simulink model "LMS_cs"  (R2023a)
settings: Solver=ode5  StartTime=0.0  StopTime=inf  FixedStep=1/200  RelTol=1e-3
PreLoadFcn:
  | mbxruntime.callbacks.PreLoadFcn(bdroot);
PostLoadFcn:
  | mbxruntime.callbacks.PostLoadFcn(bdroot);
InitFcn:
  | mbxruntime.callbacks.InitFcn(bdroot);
StartFcn:
  | mbxruntime.callbacks.StartFcn(bdroot);
StopFcn:
  | mbxruntime.callbacks.StopFcn(bdroot);
model workspace (MAT data in the model file):
  mbox_table : object (value not decoded)
  model_closed = 0
  sim_status = 0
undefined symbols (not defined in the file or in its folder): DiscIntNeverNeededParam, WheelL0, WheelL1, WheelR0, WheelR1
libraries: simulink x462, simulink_extras x117, PreScanSimulinkLibrary x33, PreScanUsefulBlocks x6, instrumentseriallib x5, simulink_need_slupdate x1
(part 66 of 68)

== system LMS_cs/BMW_X5_SUV_3/Dynamics_Simple_3D/Chassis/Bicycle_model_[XYZ]/RoadContact/RoadGeometry/zRR_lowerpenetrationdetph ==
  penetrationdepth : Inport
  position_z : Inport  Port=2
  normal_z : Inport  Port=3
  Add : Sum  Inputs=-+
  Configurable Subsystem : Subsystem  BlockChoice=Transfer Fcn  mask{ComputationMode=ComputationMode}
      mask prompts: ComputationMode "Compuation mode:"
      mask init:
      | SetComputationMode(gcb,ComputationMode);
      settings: AttributesFormatString=%<BlockChoice>  OpenFcn=BringToFront(gcb);  MemberBlocks=Discrete Transfer Fcn,Transfer Fcn
      settings: TemplateBlock=|
      | PreScanSimulinkLibrary/Configurable Subsystems/TransferFunction
      | lowerpenetrationdetph/Configurable
      | Subsystem
  Constant : Constant  Value=Inf
  Constant1 : Constant  Value=-6
  Constant2 : Constant  Value=-Inf
  Data Type Conversion : DataTypeConversion  OutDataTypeStr=double  SaturateOnIntegerOverflow=off  RndMeth=Floor
  MinMax : MinMax
  Product : Product  RndMeth=Zero
  Product1 : Product  Inputs=/*  RndMeth=Zero
  Product2 : Product  RndMeth=Zero
  Rate Limiter Dynamic : simulink/Discontinuities/Rate Limiter Dynamic
  Relational Operator : RelationalOperator  Operator===  OutDataTypeStr=boolean  InputSameDT=off
  Sum of Elements : Sum  Inputs=+
  Sum of Elements1 : Sum  Inputs=+
  Sum of Elements2 : Sum  Inputs=+
  Switch : Switch  SaturateOnIntegerOverflow=off  InputSameDT=off
  z : Outport
  wires:
  Configurable Subsystem/1(Out1) -> z/1
  Rate Limiter Dynamic/1 -> Configurable Subsystem/1(In1)
  Switch/1 -> Rate Limiter Dynamic/3
  Constant2/1 -> Switch/3
  Constant1/1 -> Switch/1
  Sum of Elements2/1 -> Switch/2
  Constant/1 -> Rate Limiter Dynamic/1
  Product1/1 -> Rate Limiter Dynamic/2
  position_z/1 -> Add/2
  Product2/1 -> Add/1
  Sum of Elements/1 -> Product1/2
  Sum of Elements1/1 -> Product1/1
  Relational Operator/1 -> Data Type Conversion/1
  Product/1 -> Sum of Elements/1
  MinMax/1 -> Relational Operator/2
  penetrationdepth/1 -> Sum of Elements2/1, Relational Operator/1, MinMax/1, Product2/1
  Add/1 -> Product/2
  normal_z/1 -> Product2/2
  Data Type Conversion/1 -> Sum of Elements1/1, Product/1

== system LMS_cs/BMW_X5_SUV_3/Dynamics_Simple_3D/Chassis/Bicycle_model_[XYZ]/RoadContact/RoadGeometry/zRR_tyreinfo ==
  In1 : Inport
  Bus Selector2 : BusSelector  OutputSignals=TireRR.cp0.penetrationdepth,TireRR.cp1.penetrationdepth,TireRR.cp2.penetrationdepth,TireRR.cp3.penetrationdepth,TireRR.cp0.position.z,TireRR.cp1.position.z,TireRR.cp2.position.z,TireRR.cp3.position.z,TireRR.cp0.normal.z,TireRR.cp1.normal.z,TireRR.cp2.normal.z,TireRR.cp3.normal.z
  Mux11 : Mux
  Mux12 : Mux
  Mux13 : Mux
  penetrationdepth : Outport
  position_z : Outport  Port=2
  normal_z : Outport  Port=3
  wires:
  Mux13/1 -> normal_z/1
  Mux12/1 -> position_z/1
  Mux11/1 -> penetrationdepth/1
  In1/1 -> Bus Selector2/1
  Bus Selector2/12 -> Mux13/4  "<z>"
  Bus Selector2/11 -> Mux13/3  "<z>"
  Bus Selector2/10 -> Mux13/2  "<z>"
  Bus Selector2/9 -> Mux13/1  "<z>"
  Bus Selector2/8 -> Mux12/4  "<z>"
  Bus Selector2/7 -> Mux12/3  "<z>"
  Bus Selector2/6 -> Mux12/2  "<z>"
  Bus Selector2/5 -> Mux12/1  "<z>"
  Bus Selector2/4 -> Mux11/4  "<penetrationdepth>"
  Bus Selector2/3 -> Mux11/3  "<penetrationdepth>"
  Bus Selector2/2 -> Mux11/2  "<penetrationdepth>"
  Bus Selector2/1 -> Mux11/1  "<penetrationdepth>"

== system LMS_cs/BMW_X5_SUV_3/Dynamics_Simple_3D/Chassis/Bicycle_model_[XYZ]/X_Motion/Max RPM and zero- velocity detection/Configurable Subsystem ==
  Step : Step  Time=0.0001  Before=1  After=0  SampleTime=0
  Out1 : Outport
  wires:
  Step/1 -> Out1/1

== system LMS_cs/BMW_X5_SUV_3/Dynamics_Simple_3D/Chassis/Bicycle_model_[XYZ]/X_Motion/Max RPM and zero- velocity detection/SR-Memory ==
  Signal : Inport
  Set : Inport  Port=2
  Reset : Inport  Port=3
  Constant : Constant  Value=0
  Detect Rise Positive : simulink/Logic and Bit Operations/Detect Rise Positive  vinit=0  OutDataTypeStr=uint8
  Detect Rise Positive1 : simulink/Logic and Bit Operations/Detect Rise Positive  vinit=0  OutDataTypeStr=uint8
  Manual Switch : ManualSwitch
  Manual Switch1 : ManualSwitch
  Switch : Switch  Criteria=u2 ~= 0  SaturateOnIntegerOverflow=off  InputSameDT=off
  Switch1 : Switch  Criteria=u2 ~= 0  SaturateOnIntegerOverflow=off  InputSameDT=off
  Unit Delay : UnitDelay  SampleTime=-1  HasFrameUpgradeWarning=on
  Out : Outport
  wires:
  Manual Switch/1 -> Switch/2
  Detect Rise Positive/1 -> Manual Switch/1
  Set/1 -> Manual Switch/2, Detect Rise Positive/1
  Unit Delay/1 -> Switch/3
  Signal/1 -> Switch/1
  Detect Rise Positive1/1 -> Manual Switch1/1
  Reset/1 -> Detect Rise Positive1/1, Manual Switch1/2
  Manual Switch1/1 -> Switch1/2
  Switch1/1 -> Out/1, Unit Delay/1
  Switch/1 -> Switch1/3
  Constant/1 -> Switch1/1

== system LMS_cs/BMW_X5_SUV_3/PreScan_Contact_Sensor/Vehicle Local to World/state2FullState/limit roll/Substitute 90 & 270 deg (and its plurals)/Angle 0-360 deg limiter ==
  Angle [deg] : Inport
  Gain : Gain  Gain=1/360
  Gain1 : Gain  Gain=360
  Rounding Function : Rounding
  Sum : Sum  Inputs=|-+
  LimAngle [deg] : Outport
  wires:
  Gain/1 -> Rounding Function/1
  Rounding Function/1 -> Gain1/1
  Gain1/1 -> Sum/1
  Angle [deg]/1 -> Gain/1, Sum/2
  Sum/1 -> LimAngle [deg]/1

== system LMS_cs/BMW_X5_SUV_4/Dynamics_Simple_3D/Chassis/Bicycle_model_[XYZ]/RoadContact/RoadGeometry/Calc_banking ==
  zi : Inport
  Constant : Constant  Value=[1, -1, 1, -1]
  Gain : Gain  Gain=1/(p.width*2)
  Product : Product  RndMeth=Zero
  Saturation : Saturate  UpperLimit=1  LowerLimit=-1
  Sum of Elements : Sum  Inputs=+
  Trigonometric Function : Trigonometry  Operator=asin
  banking : Outport
  wires:
  Saturation/1 -> Trigonometric Function/1
  zi/1 -> Product/1
  Constant/1 -> Product/2
  Product/1 -> Sum of Elements/1
  Gain/1 -> Saturation/1
  Sum of Elements/1 -> Gain/1
  Trigonometric Function/1 -> banking/1

== system LMS_cs/BMW_X5_SUV_4/Dynamics_Simple_3D/Chassis/Bicycle_model_[XYZ]/RoadContact/RoadGeometry/Calc_slope ==
  zi : Inport
  Constant : Constant  Value=[-1, -1, 1, 1]
  Gain : Gain  Gain=1/(p.l*2)
  Product : Product  RndMeth=Zero
  Saturation : Saturate  UpperLimit=1  LowerLimit=-1
  Sum of Elements : Sum  Inputs=+
  Trigonometric Function : Trigonometry  Operator=asin
  slope : Outport
  wires:
  Saturation/1 -> Trigonometric Function/1
  zi/1 -> Product/1
  Constant/1 -> Product/2
  Product/1 -> Sum of Elements/1
  Gain/1 -> Saturation/1
  Sum of Elements/1 -> Gain/1
  Trigonometric Function/1 -> slope/1

== system LMS_cs/BMW_X5_SUV_4/Dynamics_Simple_3D/Chassis/Bicycle_model_[XYZ]/RoadContact/RoadGeometry/Calc_z ==
  zi : Inport
  zC : Subsystem
  z : Outport
  wires:
  zC/1(Mean) -> z/1
  zi/1 -> zC/1(Array)

== system LMS_cs/BMW_X5_SUV_4/Dynamics_Simple_3D/Chassis/Bicycle_model_[XYZ]/RoadContact/RoadGeometry/zFL_lowerpenetrationdetph ==
  penetrationdepth : Inport
  position_z : Inport  Port=2
  normal_z : Inport  Port=3
  Add : Sum  Inputs=-+
  Configurable Subsystem : Subsystem  BlockChoice=Transfer Fcn  mask{ComputationMode=ComputationMode}
      mask prompts: ComputationMode "Compuation mode:"
      mask init:
      | SetComputationMode(gcb,ComputationMode);
      settings: AttributesFormatString=%<BlockChoice>  OpenFcn=BringToFront(gcb);  MemberBlocks=Discrete Transfer Fcn,Transfer Fcn
      settings: TemplateBlock=|
      | PreScanSimulinkLibrary/Configurable Subsystems/TransferFunction
      | lowerpenetrationdetph/Configurable
      | Subsystem
  Constant : Constant  Value=Inf
  Constant1 : Constant  Value=-6
  Constant2 : Constant  Value=-Inf
  Data Type Conversion : DataTypeConversion  OutDataTypeStr=double  SaturateOnIntegerOverflow=off  RndMeth=Floor
  MinMax : MinMax
  Product : Product  RndMeth=Zero
  Product1 : Product  Inputs=/*  RndMeth=Zero
  Product2 : Product  RndMeth=Zero
  Rate Limiter Dynamic : simulink/Discontinuities/Rate Limiter Dynamic
  Relational Operator : RelationalOperator  Operator===  OutDataTypeStr=boolean  InputSameDT=off
  Sum of Elements : Sum  Inputs=+
  Sum of Elements1 : Sum  Inputs=+
  Sum of Elements2 : Sum  Inputs=+
  Switch : Switch  SaturateOnIntegerOverflow=off  InputSameDT=off
  z : Outport
  wires:
  normal_z/1 -> Product2/2
  Add/1 -> Product/2
  penetrationdepth/1 -> Product2/1, MinMax/1, Relational Operator/1, Sum of Elements2/1
  MinMax/1 -> Relational Operator/2
  Product/1 -> Sum of Elements/1
  Relational Operator/1 -> Data Type Conversion/1
  Sum of Elements1/1 -> Product1/1
  Sum of Elements/1 -> Product1/2
  Product2/1 -> Add/1
  position_z/1 -> Add/2
  Product1/1 -> Rate Limiter Dynamic/2
  Constant/1 -> Rate Limiter Dynamic/1
  Sum of Elements2/1 -> Switch/2
  Constant1/1 -> Switch/1
  Constant2/1 -> Switch/3
  Switch/1 -> Rate Limiter Dynamic/3
  Rate Limiter Dynamic/1 -> Configurable Subsystem/1(In1)
  Configurable Subsystem/1(Out1) -> z/1
  Data Type Conversion/1 -> Product/1, Sum of Elements1/1

== system LMS_cs/BMW_X5_SUV_4/Dynamics_Simple_3D/Chassis/Bicycle_model_[XYZ]/RoadContact/RoadGeometry/zFL_tyreinfo ==
  In1 : Inport
  Bus Selector2 : BusSelector  OutputSignals=TireFL.cp0.penetrationdepth,TireFL.cp1.penetrationdepth,TireFL.cp2.penetrationdepth,TireFL.cp3.penetrationdepth,TireFL.cp0.position.z,TireFL.cp1.position.z,TireFL.cp2.position.z,TireFL.cp3.position.z,TireFL.cp0.normal.z,TireFL.cp1.normal.z,TireFL.cp2.normal.z,TireFL.cp3.normal.z
  Mux11 : Mux
  Mux12 : Mux
  Mux13 : Mux
  penetrationdepth : Outport
  position_z : Outport  Port=2
  normal_z : Outport  Port=3
  wires:
  Bus Selector2/1 -> Mux11/1  "<penetrationdepth>"
  Bus Selector2/2 -> Mux11/2  "<penetrationdepth>"
  Bus Selector2/3 -> Mux11/3  "<penetrationdepth>"
  Bus Selector2/4 -> Mux11/4  "<penetrationdepth>"
  Bus Selector2/5 -> Mux12/1  "<z>"
  Bus Selector2/6 -> Mux12/2  "<z>"
  Bus Selector2/7 -> Mux12/3  "<z>"
  Bus Selector2/8 -> Mux12/4  "<z>"
  Bus Selector2/9 -> Mux13/1  "<z>"
  Bus Selector2/10 -> Mux13/2  "<z>"
  Bus Selector2/11 -> Mux13/3  "<z>"
  Bus Selector2/12 -> Mux13/4  "<z>"
  In1/1 -> Bus Selector2/1
  Mux11/1 -> penetrationdepth/1
  Mux12/1 -> position_z/1
  Mux13/1 -> normal_z/1

== system LMS_cs/BMW_X5_SUV_4/Dynamics_Simple_3D/Chassis/Bicycle_model_[XYZ]/RoadContact/RoadGeometry/zFR_lowerpenetrationdetph ==
  penetrationdepth : Inport
  position_z : Inport  Port=2
  normal_z : Inport  Port=3
  Add : Sum  Inputs=-+
  Configurable Subsystem : Subsystem  BlockChoice=Transfer Fcn  mask{ComputationMode=ComputationMode}
      mask prompts: ComputationMode "Compuation mode:"
      mask init:
      | SetComputationMode(gcb,ComputationMode);
      settings: AttributesFormatString=%<BlockChoice>  OpenFcn=BringToFront(gcb);  MemberBlocks=Discrete Transfer Fcn,Transfer Fcn
      settings: TemplateBlock=|
      | PreScanSimulinkLibrary/Configurable Subsystems/TransferFunction
      | lowerpenetrationdetph/Configurable
      | Subsystem
  Constant : Constant  Value=Inf
  Constant1 : Constant  Value=-6
  Constant2 : Constant  Value=-Inf
  Data Type Conversion : DataTypeConversion  OutDataTypeStr=double  SaturateOnIntegerOverflow=off  RndMeth=Floor
  MinMax : MinMax
  Product : Product  RndMeth=Zero
  Product1 : Product  Inputs=/*  RndMeth=Zero
  Product2 : Product  RndMeth=Zero
  Rate Limiter Dynamic : simulink/Discontinuities/Rate Limiter Dynamic
  Relational Operator : RelationalOperator  Operator===  OutDataTypeStr=boolean  InputSameDT=off
  Sum of Elements : Sum  Inputs=+
  Sum of Elements1 : Sum  Inputs=+
  Sum of Elements2 : Sum  Inputs=+
  Switch : Switch  SaturateOnIntegerOverflow=off  InputSameDT=off
  z : Outport
  wires:
  Configurable Subsystem/1(Out1) -> z/1
  Rate Limiter Dynamic/1 -> Configurable Subsystem/1(In1)
  Switch/1 -> Rate Limiter Dynamic/3
  Constant2/1 -> Switch/3
  Constant1/1 -> Switch/1
  Sum of Elements2/1 -> Switch/2
  Constant/1 -> Rate Limiter Dynamic/1
  Product1/1 -> Rate Limiter Dynamic/2
  position_z/1 -> Add/2
  Product2/1 -> Add/1
  Sum of Elements/1 -> Product1/2
  Sum of Elements1/1 -> Product1/1
  Relational Operator/1 -> Data Type Conversion/1
  Product/1 -> Sum of Elements/1
  MinMax/1 -> Relational Operator/2
  penetrationdepth/1 -> Sum of Elements2/1, Relational Operator/1, MinMax/1, Product2/1
  Add/1 -> Product/2
  normal_z/1 -> Product2/2
  Data Type Conversion/1 -> Sum of Elements1/1, Product/1

== system LMS_cs/BMW_X5_SUV_4/Dynamics_Simple_3D/Chassis/Bicycle_model_[XYZ]/RoadContact/RoadGeometry/zFR_tyreinfo ==
  In1 : Inport
  Bus Selector2 : BusSelector  OutputSignals=TireFR.cp0.penetrationdepth,TireFR.cp1.penetrationdepth,TireFR.cp2.penetrationdepth,TireFR.cp3.penetrationdepth,TireFR.cp0.position.z,TireFR.cp1.position.z,TireFR.cp2.position.z,TireFR.cp3.position.z,TireFR.cp0.normal.z,TireFR.cp1.normal.z,TireFR.cp2.normal.z,TireFR.cp3.normal.z
  Mux11 : Mux
  Mux12 : Mux
  Mux13 : Mux
  penetrationdepth : Outport
  position_z : Outport  Port=2
  normal_z : Outport  Port=3
  wires:
  Mux13/1 -> normal_z/1
  Mux12/1 -> position_z/1
  Mux11/1 -> penetrationdepth/1
  In1/1 -> Bus Selector2/1
  Bus Selector2/12 -> Mux13/4  "<z>"
  Bus Selector2/11 -> Mux13/3  "<z>"
  Bus Selector2/10 -> Mux13/2  "<z>"
  Bus Selector2/9 -> Mux13/1  "<z>"
  Bus Selector2/8 -> Mux12/4  "<z>"
  Bus Selector2/7 -> Mux12/3  "<z>"
  Bus Selector2/6 -> Mux12/2  "<z>"
  Bus Selector2/5 -> Mux12/1  "<z>"
  Bus Selector2/4 -> Mux11/4  "<penetrationdepth>"
  Bus Selector2/3 -> Mux11/3  "<penetrationdepth>"
  Bus Selector2/2 -> Mux11/2  "<penetrationdepth>"
  Bus Selector2/1 -> Mux11/1  "<penetrationdepth>"

== system LMS_cs/BMW_X5_SUV_4/Dynamics_Simple_3D/Chassis/Bicycle_model_[XYZ]/RoadContact/RoadGeometry/zRL_lowerpenetrationdetph ==
  penetrationdepth : Inport
  position_z : Inport  Port=2
  normal_z : Inport  Port=3
  Add : Sum  Inputs=-+
  Configurable Subsystem : Subsystem  BlockChoice=Transfer Fcn  mask{ComputationMode=ComputationMode}
      mask prompts: ComputationMode "Compuation mode:"
      mask init:
      | SetComputationMode(gcb,ComputationMode);
      settings: AttributesFormatString=%<BlockChoice>  OpenFcn=BringToFront(gcb);  MemberBlocks=Discrete Transfer Fcn,Transfer Fcn
      settings: TemplateBlock=|
      | PreScanSimulinkLibrary/Configurable Subsystems/TransferFunction
      | lowerpenetrationdetph/Configurable
      | Subsystem
  Constant : Constant  Value=Inf
  Constant1 : Constant  Value=-6
  Constant2 : Constant  Value=-Inf
  Data Type Conversion : DataTypeConversion  OutDataTypeStr=double  SaturateOnIntegerOverflow=off  RndMeth=Floor
  MinMax : MinMax
  Product : Product  RndMeth=Zero
  Product1 : Product  Inputs=/*  RndMeth=Zero
  Product2 : Product  RndMeth=Zero
  Rate Limiter Dynamic : simulink/Discontinuities/Rate Limiter Dynamic
  Relational Operator : RelationalOperator  Operator===  OutDataTypeStr=boolean  InputSameDT=off
  Sum of Elements : Sum  Inputs=+
  Sum of Elements1 : Sum  Inputs=+
  Sum of Elements2 : Sum  Inputs=+
  Switch : Switch  SaturateOnIntegerOverflow=off  InputSameDT=off
  z : Outport
  wires:
  normal_z/1 -> Product2/2
  Add/1 -> Product/2
  penetrationdepth/1 -> Product2/1, MinMax/1, Relational Operator/1, Sum of Elements2/1
  MinMax/1 -> Relational Operator/2
  Product/1 -> Sum of Elements/1
  Relational Operator/1 -> Data Type Conversion/1
  Sum of Elements1/1 -> Product1/1
  Sum of Elements/1 -> Product1/2
  Product2/1 -> Add/1
  position_z/1 -> Add/2
  Product1/1 -> Rate Limiter Dynamic/2
  Constant/1 -> Rate Limiter Dynamic/1
  Sum of Elements2/1 -> Switch/2
  Constant1/1 -> Switch/1
  Constant2/1 -> Switch/3
  Switch/1 -> Rate Limiter Dynamic/3
  Rate Limiter Dynamic/1 -> Configurable Subsystem/1(In1)
  Configurable Subsystem/1(Out1) -> z/1
  Data Type Conversion/1 -> Product/1, Sum of Elements1/1

== system LMS_cs/BMW_X5_SUV_4/Dynamics_Simple_3D/Chassis/Bicycle_model_[XYZ]/RoadContact/RoadGeometry/zRL_tyreinfo ==
  In1 : Inport
  Bus Selector2 : BusSelector  OutputSignals=TireRL.cp0.penetrationdepth,TireRL.cp1.penetrationdepth,TireRL.cp2.penetrationdepth,TireRL.cp3.penetrationdepth,TireRL.cp0.position.z,TireRL.cp1.position.z,TireRL.cp2.position.z,TireRL.cp3.position.z,TireRL.cp0.normal.z,TireRL.cp1.normal.z,TireRL.cp2.normal.z,TireRL.cp3.normal.z
  Mux11 : Mux
  Mux12 : Mux
  Mux13 : Mux
  penetrationdepth : Outport
  position_z : Outport  Port=2
  normal_z : Outport  Port=3
  wires:
  Bus Selector2/1 -> Mux11/1  "<penetrationdepth>"
  Bus Selector2/2 -> Mux11/2  "<penetrationdepth>"
  Bus Selector2/3 -> Mux11/3  "<penetrationdepth>"
  Bus Selector2/4 -> Mux11/4  "<penetrationdepth>"
  Bus Selector2/5 -> Mux12/1  "<z>"
  Bus Selector2/6 -> Mux12/2  "<z>"
  Bus Selector2/7 -> Mux12/3  "<z>"
  Bus Selector2/8 -> Mux12/4  "<z>"
  Bus Selector2/9 -> Mux13/1  "<z>"
  Bus Selector2/10 -> Mux13/2  "<z>"
  Bus Selector2/11 -> Mux13/3  "<z>"
  Bus Selector2/12 -> Mux13/4  "<z>"
  In1/1 -> Bus Selector2/1
  Mux11/1 -> penetrationdepth/1
  Mux12/1 -> position_z/1
  Mux13/1 -> normal_z/1

== system LMS_cs/BMW_X5_SUV_4/Dynamics_Simple_3D/Chassis/Bicycle_model_[XYZ]/RoadContact/RoadGeometry/zRR_lowerpenetrationdetph ==
  penetrationdepth : Inport
  position_z : Inport  Port=2
  normal_z : Inport  Port=3
  Add : Sum  Inputs=-+
  Configurable Subsystem : Subsystem  BlockChoice=Transfer Fcn  mask{ComputationMode=ComputationMode}
      mask prompts: ComputationMode "Compuation mode:"
      mask init:
      | SetComputationMode(gcb,ComputationMode);
      settings: AttributesFormatString=%<BlockChoice>  OpenFcn=BringToFront(gcb);  MemberBlocks=Discrete Transfer Fcn,Transfer Fcn
      settings: TemplateBlock=|
      | PreScanSimulinkLibrary/Configurable Subsystems/TransferFunction
      | lowerpenetrationdetph/Configurable
      | Subsystem
  Constant : Constant  Value=Inf
  Constant1 : Constant  Value=-6
  Constant2 : Constant  Value=-Inf
  Data Type Conversion : DataTypeConversion  OutDataTypeStr=double  SaturateOnIntegerOverflow=off  RndMeth=Floor
  MinMax : MinMax
  Product : Product  RndMeth=Zero
  Product1 : Product  Inputs=/*  RndMeth=Zero
  Product2 : Product  RndMeth=Zero
  Rate Limiter Dynamic : simulink/Discontinuities/Rate Limiter Dynamic
  Relational Operator : RelationalOperator  Operator===  OutDataTypeStr=boolean  InputSameDT=off
  Sum of Elements : Sum  Inputs=+
  Sum of Elements1 : Sum  Inputs=+
  Sum of Elements2 : Sum  Inputs=+
  Switch : Switch  SaturateOnIntegerOverflow=off  InputSameDT=off
  z : Outport
  wires:
  Configurable Subsystem/1(Out1) -> z/1
  Rate Limiter Dynamic/1 -> Configurable Subsystem/1(In1)
  Switch/1 -> Rate Limiter Dynamic/3
  Constant2/1 -> Switch/3
  Constant1/1 -> Switch/1
  Sum of Elements2/1 -> Switch/2
  Constant/1 -> Rate Limiter Dynamic/1
  Product1/1 -> Rate Limiter Dynamic/2
  position_z/1 -> Add/2
  Product2/1 -> Add/1
  Sum of Elements/1 -> Product1/2
  Sum of Elements1/1 -> Product1/1
  Relational Operator/1 -> Data Type Conversion/1
  Product/1 -> Sum of Elements/1
  MinMax/1 -> Relational Operator/2
  penetrationdepth/1 -> Sum of Elements2/1, Relational Operator/1, MinMax/1, Product2/1
  Add/1 -> Product/2
  normal_z/1 -> Product2/2
  Data Type Conversion/1 -> Sum of Elements1/1, Product/1

== system LMS_cs/BMW_X5_SUV_4/Dynamics_Simple_3D/Chassis/Bicycle_model_[XYZ]/RoadContact/RoadGeometry/zRR_tyreinfo ==
  In1 : Inport
  Bus Selector2 : BusSelector  OutputSignals=TireRR.cp0.penetrationdepth,TireRR.cp1.penetrationdepth,TireRR.cp2.penetrationdepth,TireRR.cp3.penetrationdepth,TireRR.cp0.position.z,TireRR.cp1.position.z,TireRR.cp2.position.z,TireRR.cp3.position.z,TireRR.cp0.normal.z,TireRR.cp1.normal.z,TireRR.cp2.normal.z,TireRR.cp3.normal.z
  Mux11 : Mux
  Mux12 : Mux
  Mux13 : Mux
  penetrationdepth : Outport
  position_z : Outport  Port=2
  normal_z : Outport  Port=3
  wires:
  Mux13/1 -> normal_z/1
  Mux12/1 -> position_z/1
  Mux11/1 -> penetrationdepth/1
  In1/1 -> Bus Selector2/1
  Bus Selector2/12 -> Mux13/4  "<z>"
  Bus Selector2/11 -> Mux13/3  "<z>"
  Bus Selector2/10 -> Mux13/2  "<z>"
  Bus Selector2/9 -> Mux13/1  "<z>"
  Bus Selector2/8 -> Mux12/4  "<z>"
  Bus Selector2/7 -> Mux12/3  "<z>"
  Bus Selector2/6 -> Mux12/2  "<z>"
  Bus Selector2/5 -> Mux12/1  "<z>"
  Bus Selector2/4 -> Mux11/4  "<penetrationdepth>"
  Bus Selector2/3 -> Mux11/3  "<penetrationdepth>"
  Bus Selector2/2 -> Mux11/2  "<penetrationdepth>"
  Bus Selector2/1 -> Mux11/1  "<penetrationdepth>"

== system LMS_cs/BMW_X5_SUV_4/Dynamics_Simple_3D/Chassis/Bicycle_model_[XYZ]/X_Motion/Max RPM and zero- velocity detection/Configurable Subsystem ==
  Step : Step  Time=0.0001  Before=1  After=0  SampleTime=0
  Out1 : Outport
  wires:
  Step/1 -> Out1/1

== system LMS_cs/BMW_X5_SUV_4/Dynamics_Simple_3D/Chassis/Bicycle_model_[XYZ]/X_Motion/Max RPM and zero- velocity detection/SR-Memory ==
  Signal : Inport
  Set : Inport  Port=2
  Reset : Inport  Port=3
  Constant : Constant  Value=0
  Detect Rise Positive : simulink/Logic and Bit Operations/Detect Rise Positive  vinit=0  OutDataTypeStr=uint8
  Detect Rise Positive1 : simulink/Logic and Bit Operations/Detect Rise Positive  vinit=0  OutDataTypeStr=uint8
  Manual Switch : ManualSwitch
  Manual Switch1 : ManualSwitch
  Switch : Switch  Criteria=u2 ~= 0  SaturateOnIntegerOverflow=off  InputSameDT=off
  Switch1 : Switch  Criteria=u2 ~= 0  SaturateOnIntegerOverflow=off  InputSameDT=off
  Unit Delay : UnitDelay  SampleTime=-1  HasFrameUpgradeWarning=on
  Out : Outport
  wires:
  Manual Switch/1 -> Switch/2
  Detect Rise Positive/1 -> Manual Switch/1
  Set/1 -> Manual Switch/2, Detect Rise Positive/1
  Unit Delay/1 -> Switch/3
  Signal/1 -> Switch/1
  Detect Rise Positive1/1 -> Manual Switch1/1
  Reset/1 -> Detect Rise Positive1/1, Manual Switch1/2
  Manual Switch1/1 -> Switch1/2
  Switch1/1 -> Out/1, Unit Delay/1
  Switch/1 -> Switch1/3
  Constant/1 -> Switch1/1

== system LMS_cs/BMW_X5_SUV_4/PreScan_Contact_Sensor/Vehicle Local to World/state2FullState/limit roll/Substitute 90 & 270 deg (and its plurals)/Angle 0-360 deg limiter ==
  Angle [deg] : Inport
  Gain : Gain  Gain=1/360
  Gain1 : Gain  Gain=360
  Rounding Function : Rounding
  Sum : Sum  Inputs=|-+
  LimAngle [deg] : Outport
  wires:
  Gain/1 -> Rounding Function/1
  Rounding Function/1 -> Gain1/1
  Gain1/1 -> Sum/1
  Angle [deg]/1 -> Gain/1, Sum/2
  Sum/1 -> LimAngle [deg]/1

== system LMS_cs/BMW_X5_SUV_5/Dynamics_Simple_3D/Chassis/Bicycle_model_[XYZ]/RoadContact/RoadGeometry/Calc_banking ==
  zi : Inport
  Constant : Constant  Value=[1, -1, 1, -1]
  Gain : Gain  Gain=1/(p.width*2)
  Product : Product  RndMeth=Zero
  Saturation : Saturate  UpperLimit=1  LowerLimit=-1
  Sum of Elements : Sum  Inputs=+
  Trigonometric Function : Trigonometry  Operator=asin
  banking : Outport
  wires:
  Saturation/1 -> Trigonometric Function/1
  zi/1 -> Product/1
  Constant/1 -> Product/2
  Product/1 -> Sum of Elements/1
  Gain/1 -> Saturation/1
  Sum of Elements/1 -> Gain/1
  Trigonometric Function/1 -> banking/1

== system LMS_cs/BMW_X5_SUV_5/Dynamics_Simple_3D/Chassis/Bicycle_model_[XYZ]/RoadContact/RoadGeometry/Calc_slope ==
  zi : Inport
  Constant : Constant  Value=[-1, -1, 1, 1]
  Gain : Gain  Gain=1/(p.l*2)
  Product : Product  RndMeth=Zero
  Saturation : Saturate  UpperLimit=1  LowerLimit=-1
  Sum of Elements : Sum  Inputs=+
  Trigonometric Function : Trigonometry  Operator=asin
  slope : Outport
  wires:
  Saturation/1 -> Trigonometric Function/1
  zi/1 -> Product/1
  Constant/1 -> Product/2
  Product/1 -> Sum of Elements/1
  Gain/1 -> Saturation/1
  Sum of Elements/1 -> Gain/1
  Trigonometric Function/1 -> slope/1

== system LMS_cs/BMW_X5_SUV_5/Dynamics_Simple_3D/Chassis/Bicycle_model_[XYZ]/RoadContact/RoadGeometry/Calc_z ==
  zi : Inport
  zC : Subsystem
  z : Outport
  wires:
  zC/1(Mean) -> z/1
  zi/1 -> zC/1(Array)

== system LMS_cs/BMW_X5_SUV_5/Dynamics_Simple_3D/Chassis/Bicycle_model_[XYZ]/RoadContact/RoadGeometry/zFL_lowerpenetrationdetph ==
  penetrationdepth : Inport
  position_z : Inport  Port=2
  normal_z : Inport  Port=3
  Add : Sum  Inputs=-+
  Configurable Subsystem : Subsystem  BlockChoice=Transfer Fcn  mask{ComputationMode=ComputationMode}
      mask prompts: ComputationMode "Compuation mode:"
      mask init:
      | SetComputationMode(gcb,ComputationMode);
      settings: AttributesFormatString=%<BlockChoice>  OpenFcn=BringToFront(gcb);  MemberBlocks=Discrete Transfer Fcn,Transfer Fcn
      settings: TemplateBlock=|
      | PreScanSimulinkLibrary/Configurable Subsystems/TransferFunction
      | lowerpenetrationdetph/Configurable
      | Subsystem
  Constant : Constant  Value=Inf
  Constant1 : Constant  Value=-6
  Constant2 : Constant  Value=-Inf
  Data Type Conversion : DataTypeConversion  OutDataTypeStr=double  SaturateOnIntegerOverflow=off  RndMeth=Floor
  MinMax : MinMax
  Product : Product  RndMeth=Zero
  Product1 : Product  Inputs=/*  RndMeth=Zero
  Product2 : Product  RndMeth=Zero
  Rate Limiter Dynamic : simulink/Discontinuities/Rate Limiter Dynamic
  Relational Operator : RelationalOperator  Operator===  OutDataTypeStr=boolean  InputSameDT=off
  Sum of Elements : Sum  Inputs=+
  Sum of Elements1 : Sum  Inputs=+
  Sum of Elements2 : Sum  Inputs=+
  Switch : Switch  SaturateOnIntegerOverflow=off  InputSameDT=off
  z : Outport
  wires:
  normal_z/1 -> Product2/2
  Add/1 -> Product/2
  penetrationdepth/1 -> Product2/1, MinMax/1, Relational Operator/1, Sum of Elements2/1
  MinMax/1 -> Relational Operator/2
  Product/1 -> Sum of Elements/1
  Relational Operator/1 -> Data Type Conversion/1
  Sum of Elements1/1 -> Product1/1
  Sum of Elements/1 -> Product1/2
  Product2/1 -> Add/1
  position_z/1 -> Add/2
  Product1/1 -> Rate Limiter Dynamic/2
  Constant/1 -> Rate Limiter Dynamic/1
  Sum of Elements2/1 -> Switch/2
  Constant1/1 -> Switch/1
  Constant2/1 -> Switch/3
  Switch/1 -> Rate Limiter Dynamic/3
  Rate Limiter Dynamic/1 -> Configurable Subsystem/1(In1)
  Configurable Subsystem/1(Out1) -> z/1
  Data Type Conversion/1 -> Product/1, Sum of Elements1/1

== system LMS_cs/BMW_X5_SUV_5/Dynamics_Simple_3D/Chassis/Bicycle_model_[XYZ]/RoadContact/RoadGeometry/zFL_tyreinfo ==
  In1 : Inport
  Bus Selector2 : BusSelector  OutputSignals=TireFL.cp0.penetrationdepth,TireFL.cp1.penetrationdepth,TireFL.cp2.penetrationdepth,TireFL.cp3.penetrationdepth,TireFL.cp0.position.z,TireFL.cp1.position.z,TireFL.cp2.position.z,TireFL.cp3.position.z,TireFL.cp0.normal.z,TireFL.cp1.normal.z,TireFL.cp2.normal.z,TireFL.cp3.normal.z
  Mux11 : Mux
  Mux12 : Mux
  Mux13 : Mux
  penetrationdepth : Outport
  position_z : Outport  Port=2
  normal_z : Outport  Port=3
  wires:
  Bus Selector2/1 -> Mux11/1  "<penetrationdepth>"
  Bus Selector2/2 -> Mux11/2  "<penetrationdepth>"
  Bus Selector2/3 -> Mux11/3  "<penetrationdepth>"
  Bus Selector2/4 -> Mux11/4  "<penetrationdepth>"
  Bus Selector2/5 -> Mux12/1  "<z>"
  Bus Selector2/6 -> Mux12/2  "<z>"
  Bus Selector2/7 -> Mux12/3  "<z>"
  Bus Selector2/8 -> Mux12/4  "<z>"
  Bus Selector2/9 -> Mux13/1  "<z>"
  Bus Selector2/10 -> Mux13/2  "<z>"
  Bus Selector2/11 -> Mux13/3  "<z>"
  Bus Selector2/12 -> Mux13/4  "<z>"
  In1/1 -> Bus Selector2/1
  Mux11/1 -> penetrationdepth/1
  Mux12/1 -> position_z/1
  Mux13/1 -> normal_z/1

== system LMS_cs/BMW_X5_SUV_5/Dynamics_Simple_3D/Chassis/Bicycle_model_[XYZ]/RoadContact/RoadGeometry/zFR_lowerpenetrationdetph ==
  penetrationdepth : Inport
  position_z : Inport  Port=2
  normal_z : Inport  Port=3
  Add : Sum  Inputs=-+
  Configurable Subsystem : Subsystem  BlockChoice=Transfer Fcn  mask{ComputationMode=ComputationMode}
      mask prompts: ComputationMode "Compuation mode:"
      mask init:
      | SetComputationMode(gcb,ComputationMode);
      settings: AttributesFormatString=%<BlockChoice>  OpenFcn=BringToFront(gcb);  MemberBlocks=Discrete Transfer Fcn,Transfer Fcn
      settings: TemplateBlock=|
      | PreScanSimulinkLibrary/Configurable Subsystems/TransferFunction
      | lowerpenetrationdetph/Configurable
      | Subsystem
  Constant : Constant  Value=Inf
  Constant1 : Constant  Value=-6
  Constant2 : Constant  Value=-Inf
  Data Type Conversion : DataTypeConversion  OutDataTypeStr=double  SaturateOnIntegerOverflow=off  RndMeth=Floor
  MinMax : MinMax
  Product : Product  RndMeth=Zero
  Product1 : Product  Inputs=/*  RndMeth=Zero
  Product2 : Product  RndMeth=Zero
  Rate Limiter Dynamic : simulink/Discontinuities/Rate Limiter Dynamic
  Relational Operator : RelationalOperator  Operator===  OutDataTypeStr=boolean  InputSameDT=off
  Sum of Elements : Sum  Inputs=+
  Sum of Elements1 : Sum  Inputs=+
  Sum of Elements2 : Sum  Inputs=+
  Switch : Switch  SaturateOnIntegerOverflow=off  InputSameDT=off
  z : Outport
  wires:
  Configurable Subsystem/1(Out1) -> z/1
  Rate Limiter Dynamic/1 -> Configurable Subsystem/1(In1)
  Switch/1 -> Rate Limiter Dynamic/3
  Constant2/1 -> Switch/3
  Constant1/1 -> Switch/1
  Sum of Elements2/1 -> Switch/2
  Constant/1 -> Rate Limiter Dynamic/1
  Product1/1 -> Rate Limiter Dynamic/2
  position_z/1 -> Add/2
  Product2/1 -> Add/1
  Sum of Elements/1 -> Product1/2
  Sum of Elements1/1 -> Product1/1
  Relational Operator/1 -> Data Type Conversion/1
  Product/1 -> Sum of Elements/1
  MinMax/1 -> Relational Operator/2
  penetrationdepth/1 -> Sum of Elements2/1, Relational Operator/1, MinMax/1, Product2/1
  Add/1 -> Product/2
  normal_z/1 -> Product2/2
  Data Type Conversion/1 -> Sum of Elements1/1, Product/1

== system LMS_cs/BMW_X5_SUV_5/Dynamics_Simple_3D/Chassis/Bicycle_model_[XYZ]/RoadContact/RoadGeometry/zFR_tyreinfo ==
  In1 : Inport
  Bus Selector2 : BusSelector  OutputSignals=TireFR.cp0.penetrationdepth,TireFR.cp1.penetrationdepth,TireFR.cp2.penetrationdepth,TireFR.cp3.penetrationdepth,TireFR.cp0.position.z,TireFR.cp1.position.z,TireFR.cp2.position.z,TireFR.cp3.position.z,TireFR.cp0.normal.z,TireFR.cp1.normal.z,TireFR.cp2.normal.z,TireFR.cp3.normal.z
  Mux11 : Mux
  Mux12 : Mux
  Mux13 : Mux
  penetrationdepth : Outport
  position_z : Outport  Port=2
  normal_z : Outport  Port=3
  wires:
  Mux13/1 -> normal_z/1
  Mux12/1 -> position_z/1
  Mux11/1 -> penetrationdepth/1
  In1/1 -> Bus Selector2/1
  Bus Selector2/12 -> Mux13/4  "<z>"
  Bus Selector2/11 -> Mux13/3  "<z>"
  Bus Selector2/10 -> Mux13/2  "<z>"
  Bus Selector2/9 -> Mux13/1  "<z>"
  Bus Selector2/8 -> Mux12/4  "<z>"
  Bus Selector2/7 -> Mux12/3  "<z>"
  Bus Selector2/6 -> Mux12/2  "<z>"
  Bus Selector2/5 -> Mux12/1  "<z>"
  Bus Selector2/4 -> Mux11/4  "<penetrationdepth>"
  Bus Selector2/3 -> Mux11/3  "<penetrationdepth>"
  Bus Selector2/2 -> Mux11/2  "<penetrationdepth>"
  Bus Selector2/1 -> Mux11/1  "<penetrationdepth>"

== system LMS_cs/BMW_X5_SUV_5/Dynamics_Simple_3D/Chassis/Bicycle_model_[XYZ]/RoadContact/RoadGeometry/zRL_lowerpenetrationdetph ==
  penetrationdepth : Inport
  position_z : Inport  Port=2
  normal_z : Inport  Port=3
  Add : Sum  Inputs=-+
  Configurable Subsystem : Subsystem  BlockChoice=Transfer Fcn  mask{ComputationMode=ComputationMode}
      mask prompts: ComputationMode "Compuation mode:"
      mask init:
      | SetComputationMode(gcb,ComputationMode);
      settings: AttributesFormatString=%<BlockChoice>  OpenFcn=BringToFront(gcb);  MemberBlocks=Discrete Transfer Fcn,Transfer Fcn
      settings: TemplateBlock=|
      | PreScanSimulinkLibrary/Configurable Subsystems/TransferFunction
      | lowerpenetrationdetph/Configurable
      | Subsystem
  Constant : Constant  Value=Inf
  Constant1 : Constant  Value=-6
  Constant2 : Constant  Value=-Inf
  Data Type Conversion : DataTypeConversion  OutDataTypeStr=double  SaturateOnIntegerOverflow=off  RndMeth=Floor
  MinMax : MinMax
  Product : Product  RndMeth=Zero
  Product1 : Product  Inputs=/*  RndMeth=Zero
  Product2 : Product  RndMeth=Zero
  Rate Limiter Dynamic : simulink/Discontinuities/Rate Limiter Dynamic
  Relational Operator : RelationalOperator  Operator===  OutDataTypeStr=boolean  InputSameDT=off
  Sum of Elements : Sum  Inputs=+
  Sum of Elements1 : Sum  Inputs=+
  Sum of Elements2 : Sum  Inputs=+
  Switch : Switch  SaturateOnIntegerOverflow=off  InputSameDT=off
  z : Outport
  wires:
  normal_z/1 -> Product2/2
  Add/1 -> Product/2
  penetrationdepth/1 -> Product2/1, MinMax/1, Relational Operator/1, Sum of Elements2/1
  MinMax/1 -> Relational Operator/2
  Product/1 -> Sum of Elements/1
  Relational Operator/1 -> Data Type Conversion/1
  Sum of Elements1/1 -> Product1/1
  Sum of Elements/1 -> Product1/2
  Product2/1 -> Add/1
  position_z/1 -> Add/2
  Product1/1 -> Rate Limiter Dynamic/2
  Constant/1 -> Rate Limiter Dynamic/1
  Sum of Elements2/1 -> Switch/2
  Constant1/1 -> Switch/1
  Constant2/1 -> Switch/3
  Switch/1 -> Rate Limiter Dynamic/3
  Rate Limiter Dynamic/1 -> Configurable Subsystem/1(In1)
  Configurable Subsystem/1(Out1) -> z/1
  Data Type Conversion/1 -> Product/1, Sum of Elements1/1

== system LMS_cs/BMW_X5_SUV_5/Dynamics_Simple_3D/Chassis/Bicycle_model_[XYZ]/RoadContact/RoadGeometry/zRL_tyreinfo ==
  In1 : Inport
  Bus Selector2 : BusSelector  OutputSignals=TireRL.cp0.penetrationdepth,TireRL.cp1.penetrationdepth,TireRL.cp2.penetrationdepth,TireRL.cp3.penetrationdepth,TireRL.cp0.position.z,TireRL.cp1.position.z,TireRL.cp2.position.z,TireRL.cp3.position.z,TireRL.cp0.normal.z,TireRL.cp1.normal.z,TireRL.cp2.normal.z,TireRL.cp3.normal.z
  Mux11 : Mux
  Mux12 : Mux
  Mux13 : Mux
  penetrationdepth : Outport
  position_z : Outport  Port=2
  normal_z : Outport  Port=3
  wires:
  Bus Selector2/1 -> Mux11/1  "<penetrationdepth>"
  Bus Selector2/2 -> Mux11/2  "<penetrationdepth>"
  Bus Selector2/3 -> Mux11/3  "<penetrationdepth>"
  Bus Selector2/4 -> Mux11/4  "<penetrationdepth>"
  Bus Selector2/5 -> Mux12/1  "<z>"
  Bus Selector2/6 -> Mux12/2  "<z>"
  Bus Selector2/7 -> Mux12/3  "<z>"
  Bus Selector2/8 -> Mux12/4  "<z>"
  Bus Selector2/9 -> Mux13/1  "<z>"
  Bus Selector2/10 -> Mux13/2  "<z>"
  Bus Selector2/11 -> Mux13/3  "<z>"
  Bus Selector2/12 -> Mux13/4  "<z>"
  In1/1 -> Bus Selector2/1
  Mux11/1 -> penetrationdepth/1
  Mux12/1 -> position_z/1
  Mux13/1 -> normal_z/1

== system LMS_cs/BMW_X5_SUV_5/Dynamics_Simple_3D/Chassis/Bicycle_model_[XYZ]/RoadContact/RoadGeometry/zRR_lowerpenetrationdetph ==
  penetrationdepth : Inport
  position_z : Inport  Port=2
  normal_z : Inport  Port=3
  Add : Sum  Inputs=-+
  Configurable Subsystem : Subsystem  BlockChoice=Transfer Fcn  mask{ComputationMode=ComputationMode}
      mask prompts: ComputationMode "Compuation mode:"
      mask init:
      | SetComputationMode(gcb,ComputationMode);
      settings: AttributesFormatString=%<BlockChoice>  OpenFcn=BringToFront(gcb);  MemberBlocks=Discrete Transfer Fcn,Transfer Fcn
      settings: TemplateBlock=|
      | PreScanSimulinkLibrary/Configurable Subsystems/TransferFunction
      | lowerpenetrationdetph/Configurable
      | Subsystem
  Constant : Constant  Value=Inf
  Constant1 : Constant  Value=-6
  Constant2 : Constant  Value=-Inf
  Data Type Conversion : DataTypeConversion  OutDataTypeStr=double  SaturateOnIntegerOverflow=off  RndMeth=Floor
  MinMax : MinMax
  Product : Product  RndMeth=Zero
  Product1 : Product  Inputs=/*  RndMeth=Zero
  Product2 : Product  RndMeth=Zero
  Rate Limiter Dynamic : simulink/Discontinuities/Rate Limiter Dynamic
  Relational Operator : RelationalOperator  Operator===  OutDataTypeStr=boolean  InputSameDT=off
  Sum of Elements : Sum  Inputs=+
  Sum of Elements1 : Sum  Inputs=+
  Sum of Elements2 : Sum  Inputs=+
  Switch : Switch  SaturateOnIntegerOverflow=off  InputSameDT=off
  z : Outport
  wires:
  Configurable Subsystem/1(Out1) -> z/1
  Rate Limiter Dynamic/1 -> Configurable Subsystem/1(In1)
  Switch/1 -> Rate Limiter Dynamic/3
  Constant2/1 -> Switch/3
  Constant1/1 -> Switch/1
  Sum of Elements2/1 -> Switch/2
  Constant/1 -> Rate Limiter Dynamic/1
  Product1/1 -> Rate Limiter Dynamic/2
  position_z/1 -> Add/2
  Product2/1 -> Add/1
  Sum of Elements/1 -> Product1/2
  Sum of Elements1/1 -> Product1/1
  Relational Operator/1 -> Data Type Conversion/1
  Product/1 -> Sum of Elements/1
  MinMax/1 -> Relational Operator/2
  penetrationdepth/1 -> Sum of Elements2/1, Relational Operator/1, MinMax/1, Product2/1
  Add/1 -> Product/2
  normal_z/1 -> Product2/2
  Data Type Conversion/1 -> Sum of Elements1/1, Product/1

== system LMS_cs/BMW_X5_SUV_5/Dynamics_Simple_3D/Chassis/Bicycle_model_[XYZ]/RoadContact/RoadGeometry/zRR_tyreinfo ==
  In1 : Inport
  Bus Selector2 : BusSelector  OutputSignals=TireRR.cp0.penetrationdepth,TireRR.cp1.penetrationdepth,TireRR.cp2.penetrationdepth,TireRR.cp3.penetrationdepth,TireRR.cp0.position.z,TireRR.cp1.position.z,TireRR.cp2.position.z,TireRR.cp3.position.z,TireRR.cp0.normal.z,TireRR.cp1.normal.z,TireRR.cp2.normal.z,TireRR.cp3.normal.z
  Mux11 : Mux
  Mux12 : Mux
  Mux13 : Mux
  penetrationdepth : Outport
  position_z : Outport  Port=2
  normal_z : Outport  Port=3
  wires:
  Mux13/1 -> normal_z/1
  Mux12/1 -> position_z/1
  Mux11/1 -> penetrationdepth/1
  In1/1 -> Bus Selector2/1
  Bus Selector2/12 -> Mux13/4  "<z>"
  Bus Selector2/11 -> Mux13/3  "<z>"
  Bus Selector2/10 -> Mux13/2  "<z>"
  Bus Selector2/9 -> Mux13/1  "<z>"
  Bus Selector2/8 -> Mux12/4  "<z>"
  Bus Selector2/7 -> Mux12/3  "<z>"
  Bus Selector2/6 -> Mux12/2  "<z>"
  Bus Selector2/5 -> Mux12/1  "<z>"
  Bus Selector2/4 -> Mux11/4  "<penetrationdepth>"
  Bus Selector2/3 -> Mux11/3  "<penetrationdepth>"
  Bus Selector2/2 -> Mux11/2  "<penetrationdepth>"
  Bus Selector2/1 -> Mux11/1  "<penetrationdepth>"

== system LMS_cs/BMW_X5_SUV_5/Dynamics_Simple_3D/Chassis/Bicycle_model_[XYZ]/X_Motion/Max RPM and zero- velocity detection/Configurable Subsystem ==
  Step : Step  Time=0.0001  Before=1  After=0  SampleTime=0
  Out1 : Outport
  wires:
  Step/1 -> Out1/1

== system LMS_cs/BMW_X5_SUV_5/Dynamics_Simple_3D/Chassis/Bicycle_model_[XYZ]/X_Motion/Max RPM and zero- velocity detection/SR-Memory ==
  Signal : Inport
  Set : Inport  Port=2
  Reset : Inport  Port=3
  Constant : Constant  Value=0
  Detect Rise Positive : simulink/Logic and Bit Operations/Detect Rise Positive  vinit=0  OutDataTypeStr=uint8
  Detect Rise Positive1 : simulink/Logic and Bit Operations/Detect Rise Positive  vinit=0  OutDataTypeStr=uint8
  Manual Switch : ManualSwitch
  Manual Switch1 : ManualSwitch
  Switch : Switch  Criteria=u2 ~= 0  SaturateOnIntegerOverflow=off  InputSameDT=off
  Switch1 : Switch  Criteria=u2 ~= 0  SaturateOnIntegerOverflow=off  InputSameDT=off
  Unit Delay : UnitDelay  SampleTime=-1  HasFrameUpgradeWarning=on
  Out : Outport
  wires:
  Manual Switch/1 -> Switch/2
  Detect Rise Positive/1 -> Manual Switch/1
  Set/1 -> Manual Switch/2, Detect Rise Positive/1
  Unit Delay/1 -> Switch/3
  Signal/1 -> Switch/1
  Detect Rise Positive1/1 -> Manual Switch1/1
  Reset/1 -> Detect Rise Positive1/1, Manual Switch1/2
  Manual Switch1/1 -> Switch1/2
  Switch1/1 -> Out/1, Unit Delay/1
  Switch/1 -> Switch1/3
  Constant/1 -> Switch1/1

== system LMS_cs/BMW_X5_SUV_5/PreScan_Contact_Sensor/Vehicle Local to World/state2FullState/limit roll/Substitute 90 & 270 deg (and its plurals)/Angle 0-360 deg limiter ==
  Angle [deg] : Inport
  Gain : Gain  Gain=1/360
  Gain1 : Gain  Gain=360
  Rounding Function : Rounding
  Sum : Sum  Inputs=|-+
  LimAngle [deg] : Outport
  wires:
  Gain/1 -> Rounding Function/1
  Rounding Function/1 -> Gain1/1
  Gain1/1 -> Sum/1
  Angle [deg]/1 -> Gain/1, Sum/2
  Sum/1 -> LimAngle [deg]/1

== system LMS_cs/BMW_X5_SUV_6/Dynamics_Simple_3D/Chassis/Bicycle_model_[XYZ]/RoadContact/RoadGeometry/Calc_banking ==
  zi : Inport
  Constant : Constant  Value=[1, -1, 1, -1]
  Gain : Gain  Gain=1/(p.width*2)
  Product : Product  RndMeth=Zero
  Saturation : Saturate  UpperLimit=1  LowerLimit=-1
  Sum of Elements : Sum  Inputs=+
  Trigonometric Function : Trigonometry  Operator=asin
  banking : Outport
  wires:
  Saturation/1 -> Trigonometric Function/1
  zi/1 -> Product/1
  Constant/1 -> Product/2
  Product/1 -> Sum of Elements/1
  Gain/1 -> Saturation/1
  Sum of Elements/1 -> Gain/1
  Trigonometric Function/1 -> banking/1

== system LMS_cs/BMW_X5_SUV_6/Dynamics_Simple_3D/Chassis/Bicycle_model_[XYZ]/RoadContact/RoadGeometry/Calc_slope ==
  zi : Inport
  Constant : Constant  Value=[-1, -1, 1, 1]
  Gain : Gain  Gain=1/(p.l*2)
  Product : Product  RndMeth=Zero
  Saturation : Saturate  UpperLimit=1  LowerLimit=-1
  Sum of Elements : Sum  Inputs=+
  Trigonometric Function : Trigonometry  Operator=asin
  slope : Outport
  wires:
  Saturation/1 -> Trigonometric Function/1
  zi/1 -> Product/1
  Constant/1 -> Product/2
  Product/1 -> Sum of Elements/1
  Gain/1 -> Saturation/1
  Sum of Elements/1 -> Gain/1
  Trigonometric Function/1 -> slope/1

== system LMS_cs/BMW_X5_SUV_6/Dynamics_Simple_3D/Chassis/Bicycle_model_[XYZ]/RoadContact/RoadGeometry/Calc_z ==
  zi : Inport
  zC : Subsystem
  z : Outport
  wires:
  zC/1(Mean) -> z/1
  zi/1 -> zC/1(Array)

== system LMS_cs/BMW_X5_SUV_6/Dynamics_Simple_3D/Chassis/Bicycle_model_[XYZ]/RoadContact/RoadGeometry/zFL_lowerpenetrationdetph ==
  penetrationdepth : Inport
  position_z : Inport  Port=2
  normal_z : Inport  Port=3
  Add : Sum  Inputs=-+
  Configurable Subsystem : Subsystem  BlockChoice=Transfer Fcn  mask{ComputationMode=ComputationMode}
      mask prompts: ComputationMode "Compuation mode:"
      mask init:
      | SetComputationMode(gcb,ComputationMode);
      settings: AttributesFormatString=%<BlockChoice>  OpenFcn=BringToFront(gcb);  MemberBlocks=Discrete Transfer Fcn,Transfer Fcn
      settings: TemplateBlock=|
      | PreScanSimulinkLibrary/Configurable Subsystems/TransferFunction
      | lowerpenetrationdetph/Configurable
      | Subsystem
  Constant : Constant  Value=Inf
  Constant1 : Constant  Value=-6
  Constant2 : Constant  Value=-Inf
  Data Type Conversion : DataTypeConversion  OutDataTypeStr=double  SaturateOnIntegerOverflow=off  RndMeth=Floor
  MinMax : MinMax
  Product : Product  RndMeth=Zero
  Product1 : Product  Inputs=/*  RndMeth=Zero
  Product2 : Product  RndMeth=Zero
  Rate Limiter Dynamic : simulink/Discontinuities/Rate Limiter Dynamic
  Relational Operator : RelationalOperator  Operator===  OutDataTypeStr=boolean  InputSameDT=off
  Sum of Elements : Sum  Inputs=+
  Sum of Elements1 : Sum  Inputs=+
  Sum of Elements2 : Sum  Inputs=+
  Switch : Switch  SaturateOnIntegerOverflow=off  InputSameDT=off
  z : Outport
  wires:
  normal_z/1 -> Product2/2
  Add/1 -> Product/2
  penetrationdepth/1 -> Product2/1, MinMax/1, Relational Operator/1, Sum of Elements2/1
  MinMax/1 -> Relational Operator/2
  Product/1 -> Sum of Elements/1
  Relational Operator/1 -> Data Type Conversion/1
  Sum of Elements1/1 -> Product1/1
  Sum of Elements/1 -> Product1/2
  Product2/1 -> Add/1
  position_z/1 -> Add/2
  Product1/1 -> Rate Limiter Dynamic/2
  Constant/1 -> Rate Limiter Dynamic/1
  Sum of Elements2/1 -> Switch/2
  Constant1/1 -> Switch/1
  Constant2/1 -> Switch/3
  Switch/1 -> Rate Limiter Dynamic/3
  Rate Limiter Dynamic/1 -> Configurable Subsystem/1(In1)
  Configurable Subsystem/1(Out1) -> z/1
  Data Type Conversion/1 -> Product/1, Sum of Elements1/1

== system LMS_cs/BMW_X5_SUV_6/Dynamics_Simple_3D/Chassis/Bicycle_model_[XYZ]/RoadContact/RoadGeometry/zFL_tyreinfo ==
  In1 : Inport
  Bus Selector2 : BusSelector  OutputSignals=TireFL.cp0.penetrationdepth,TireFL.cp1.penetrationdepth,TireFL.cp2.penetrationdepth,TireFL.cp3.penetrationdepth,TireFL.cp0.position.z,TireFL.cp1.position.z,TireFL.cp2.position.z,TireFL.cp3.position.z,TireFL.cp0.normal.z,TireFL.cp1.normal.z,TireFL.cp2.normal.z,TireFL.cp3.normal.z
  Mux11 : Mux
  Mux12 : Mux
  Mux13 : Mux
  penetrationdepth : Outport
  position_z : Outport  Port=2
  normal_z : Outport  Port=3
  wires:
  Bus Selector2/1 -> Mux11/1  "<penetrationdepth>"
  Bus Selector2/2 -> Mux11/2  "<penetrationdepth>"
  Bus Selector2/3 -> Mux11/3  "<penetrationdepth>"
  Bus Selector2/4 -> Mux11/4  "<penetrationdepth>"
  Bus Selector2/5 -> Mux12/1  "<z>"
  Bus Selector2/6 -> Mux12/2  "<z>"
  Bus Selector2/7 -> Mux12/3  "<z>"
  Bus Selector2/8 -> Mux12/4  "<z>"
  Bus Selector2/9 -> Mux13/1  "<z>"
  Bus Selector2/10 -> Mux13/2  "<z>"
  Bus Selector2/11 -> Mux13/3  "<z>"
  Bus Selector2/12 -> Mux13/4  "<z>"
  In1/1 -> Bus Selector2/1
  Mux11/1 -> penetrationdepth/1
  Mux12/1 -> position_z/1
  Mux13/1 -> normal_z/1

== system LMS_cs/BMW_X5_SUV_6/Dynamics_Simple_3D/Chassis/Bicycle_model_[XYZ]/RoadContact/RoadGeometry/zFR_lowerpenetrationdetph ==
  penetrationdepth : Inport
  position_z : Inport  Port=2
  normal_z : Inport  Port=3
  Add : Sum  Inputs=-+
  Configurable Subsystem : Subsystem  BlockChoice=Transfer Fcn  mask{ComputationMode=ComputationMode}
      mask prompts: ComputationMode "Compuation mode:"
      mask init:
      | SetComputationMode(gcb,ComputationMode);
      settings: AttributesFormatString=%<BlockChoice>  OpenFcn=BringToFront(gcb);  MemberBlocks=Discrete Transfer Fcn,Transfer Fcn
      settings: TemplateBlock=|
      | PreScanSimulinkLibrary/Configurable Subsystems/TransferFunction
      | lowerpenetrationdetph/Configurable
      | Subsystem
  Constant : Constant  Value=Inf
  Constant1 : Constant  Value=-6
  Constant2 : Constant  Value=-Inf
  Data Type Conversion : DataTypeConversion  OutDataTypeStr=double  SaturateOnIntegerOverflow=off  RndMeth=Floor
  MinMax : MinMax
  Product : Product  RndMeth=Zero
  Product1 : Product  Inputs=/*  RndMeth=Zero
  Product2 : Product  RndMeth=Zero
  Rate Limiter Dynamic : simulink/Discontinuities/Rate Limiter Dynamic
  Relational Operator : RelationalOperator  Operator===  OutDataTypeStr=boolean  InputSameDT=off
  Sum of Elements : Sum  Inputs=+
  Sum of Elements1 : Sum  Inputs=+
  Sum of Elements2 : Sum  Inputs=+
  Switch : Switch  SaturateOnIntegerOverflow=off  InputSameDT=off
  z : Outport
  wires:
  Configurable Subsystem/1(Out1) -> z/1
  Rate Limiter Dynamic/1 -> Configurable Subsystem/1(In1)
  Switch/1 -> Rate Limiter Dynamic/3
  Constant2/1 -> Switch/3
  Constant1/1 -> Switch/1
  Sum of Elements2/1 -> Switch/2
  Constant/1 -> Rate Limiter Dynamic/1
  Product1/1 -> Rate Limiter Dynamic/2
  position_z/1 -> Add/2
  Product2/1 -> Add/1
  Sum of Elements/1 -> Product1/2
  Sum of Elements1/1 -> Product1/1
  Relational Operator/1 -> Data Type Conversion/1
  Product/1 -> Sum of Elements/1
  MinMax/1 -> Relational Operator/2
  penetrationdepth/1 -> Sum of Elements2/1, Relational Operator/1, MinMax/1, Product2/1
  Add/1 -> Product/2
  normal_z/1 -> Product2/2
  Data Type Conversion/1 -> Sum of Elements1/1, Product/1

== system LMS_cs/BMW_X5_SUV_6/Dynamics_Simple_3D/Chassis/Bicycle_model_[XYZ]/RoadContact/RoadGeometry/zFR_tyreinfo ==
  In1 : Inport
  Bus Selector2 : BusSelector  OutputSignals=TireFR.cp0.penetrationdepth,TireFR.cp1.penetrationdepth,TireFR.cp2.penetrationdepth,TireFR.cp3.penetrationdepth,TireFR.cp0.position.z,TireFR.cp1.position.z,TireFR.cp2.position.z,TireFR.cp3.position.z,TireFR.cp0.normal.z,TireFR.cp1.normal.z,TireFR.cp2.normal.z,TireFR.cp3.normal.z
  Mux11 : Mux
  Mux12 : Mux
  Mux13 : Mux
  penetrationdepth : Outport
  position_z : Outport  Port=2
  normal_z : Outport  Port=3
  wires:
  Mux13/1 -> normal_z/1
  Mux12/1 -> position_z/1
  Mux11/1 -> penetrationdepth/1
  In1/1 -> Bus Selector2/1
  Bus Selector2/12 -> Mux13/4  "<z>"
  Bus Selector2/11 -> Mux13/3  "<z>"
  Bus Selector2/10 -> Mux13/2  "<z>"
  Bus Selector2/9 -> Mux13/1  "<z>"
  Bus Selector2/8 -> Mux12/4  "<z>"
  Bus Selector2/7 -> Mux12/3  "<z>"
  Bus Selector2/6 -> Mux12/2  "<z>"
  Bus Selector2/5 -> Mux12/1  "<z>"
  Bus Selector2/4 -> Mux11/4  "<penetrationdepth>"
  Bus Selector2/3 -> Mux11/3  "<penetrationdepth>"
  Bus Selector2/2 -> Mux11/2  "<penetrationdepth>"
  Bus Selector2/1 -> Mux11/1  "<penetrationdepth>"
